simulink model "Scrambler_remoto"  (R2013a)
settings: Solver=FixedStepDiscrete  StartTime=0.0  StopTime=10.0  RelTol=1e-3
settings Model: Creator=Élio  LastModifiedBy=Élio
settings OptimizationCC: InlineParams=on

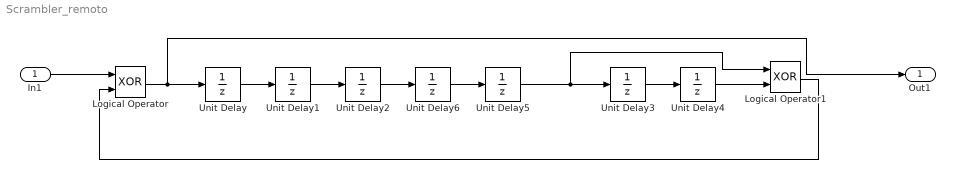
== system Scrambler_remoto ==
  In1 : Inport
  Logical Operator : Logic  Operator=XOR  AllPortsSameDT=off  OutDataTypeStr=fixdt(1,16)
  Logical Operator1 : Logic  Operator=XOR  AllPortsSameDT=off  OutDataTypeStr=fixdt(1,16)
  Unit Delay{,1..6} (7 alike) : UnitDelay  SampleTime=-1
  Out1 : Outport
  wires:
  Unit Delay/1 -> Unit Delay1/1
  Unit Delay1/1 -> Unit Delay2/1
  Unit Delay3/1 -> Unit Delay4/1
  Unit Delay4/1 -> Logical Operator1/2
  Logical Operator1/1 -> Logical Operator/2
  Logical Operator/1 -> Out1/1, Unit Delay/1
  In1/1 -> Logical Operator/1
  Unit Delay2/1 -> Unit Delay6/1
  Unit Delay6/1 -> Unit Delay5/1
  Unit Delay5/1 -> Logical Operator1/1, Unit Delay3/1
